simulink model "DIFFERENCE_EQUATION_FILTER_4"  (R2020b)
settings: Solver=VariableStepAuto  StartTime=0.0  StopTime=10  RelTol=1e-3
undefined symbols (not defined in the file): a0, a1, b1, b2
settings Model: DataDictionary=data_dictionary_for_probl4.sldd  Creator=intel  LastModifiedBy=intel

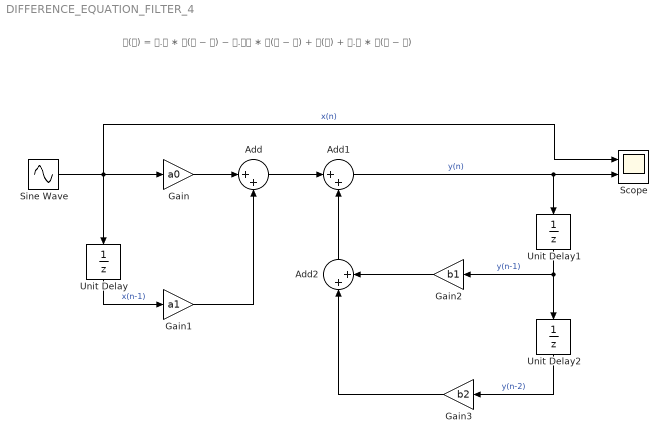
== system DIFFERENCE_EQUATION_FILTER_4 ==
  note: 𝐲(𝐧) = 𝟎.𝟓 ∗ 𝐲(𝐧 − 𝟏) − 𝟎.𝟐𝟓 ∗ 𝐲(𝐧 − 𝟐) + 𝐱(𝐧) + 𝟎.𝟒 ∗ 𝐱(𝐧 − 𝟏)
  Add : Sum  Inputs=|++
  Add1 : Sum  Inputs=|++
  Add2 : Sum  Inputs=|++
  Gain : Gain  Gain=a0
  Gain1 : Gain  Gain=a1
  Gain2 : Gain  Gain=b1
  Gain3 : Gain  Gain=b2
  Scope : Scope  NumInputPorts=2
  Sine Wave : Sin  SampleTime=0
  Unit Delay : UnitDelay  SampleTime=-1  HasFrameUpgradeWarning=on
  Unit Delay1 : UnitDelay  SampleTime=-1  HasFrameUpgradeWarning=on
  Unit Delay2 : UnitDelay  SampleTime=-1  HasFrameUpgradeWarning=on
  wires:
  Sine Wave/1 -> Unit Delay/1, Scope/1, Gain/1  "x(n)"
  Gain/1 -> Add/1
  Gain1/1 -> Add/2
  Add/1 -> Add1/1
  Add2/1 -> Add1/2
  Unit Delay/1 -> Gain1/1  "x(n-1)"
  Gain2/1 -> Add2/2
  Gain3/1 -> Add2/1
  Add1/1 -> Unit Delay1/1, Scope/2  "y(n)"
  Unit Delay1/1 -> Unit Delay2/1, Gain2/1  "y(n-1)"
  Unit Delay2/1 -> Gain3/1  "y(n-2)"
